simulink model "RR_Aero_Forces"  (R2023b)
settings: Solver=ode45  StartTime=0.0  StopTime=10.0  RelTol=1e-3
values from neighbouring files (symbols this model uses):
  RR_Aero_Aoa = [-40 -20 -10 -5 0 5 10 20 40]    [RR.mat]    (also in aero.m = [-40.0, -20.0, -10.0, -5.0, 0.0, 5.0, 10.0, 20.0, 40.0])
  RR_Aero_CD = [0.682566420597 0.618503123563 0.559439658146 0.524132967178 0.485737326161 0.447874599784 0.410140259349 0.344355457301 0.271986762452 0.285740001736 0.220860646778 0.173194791928 ... (405 elements, 9x9x5)]    [RR.mat]    (also in aero.m = flip([0.271986762452 0.048967807354 0.024623797928 0.0311930)
  RR_Aero_CL = [-1.32787481318 -1.28000797148 -1.22978921447 -1.19580936529 -1.15925228344 -1.11732991534 -1.07321949156 -0.982213833372 -0.840672452343 -1.01110225062 -0.901800471345 -0.804191382013 ... (405 elements, 9x9x5)]    [RR.mat]    (also in aero.m = flip([-0.840672452343 -0.271053660865 0.064194032020 0.23384)
  RR_Aero_CMy = [0.261776710059 0.227892723507 0.194122810948 0.17203964717 0.149197278338 0.123782621534 0.09809104025 0.048156954183 -0.022673613914 0.230490752369 0.172298182326 0.122095577928 ... (405 elements, 9x9x5)]    [RR.mat]    (also in aero.m = flip([-0.022673613914 -0.123256713392 -0.153636001960 -0.164)
  RR_Aero_Elevons = [-40 -20 -10 -5 0 5 10 20 40]    [RR.mat]    (also in aero.m = [-40.0, -20.0, -10.0, -5.0, 0.0, 5.0, 10.0, 20.0, 40.0])
  RR_Aero_Mach = [0.01 0.1 0.2 0.5 0.9]    [RR.mat]    (also in aero.m = [0.01, 0.1, 0.2, 0.5, 0.9])
  RR_Span = 3.6    [RR.mat]
  RR_X_CG = 0.732425    [RR.mat]
  RR_X_NP = 0.9170209    [RR.mat]
libraries: aerolibasang x2, aerolibadyn x1, aerolibatmos2 x1
settings Model: Creator=jrighetti  LastModifiedBy=jrighetti

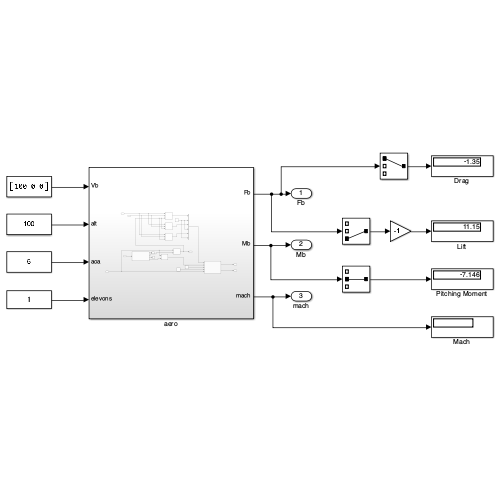
[thumbnail: Simulink's stored preview of the top-level diagram]
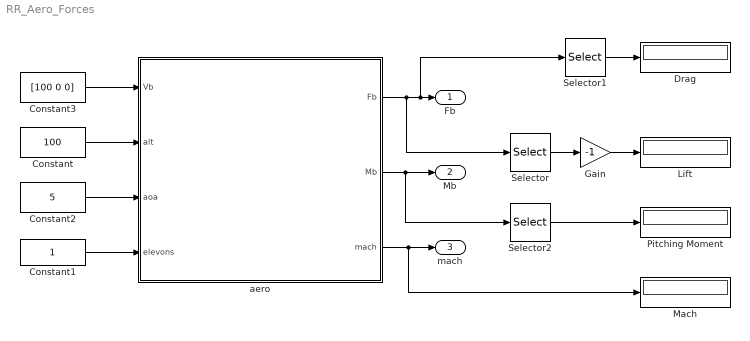
== system RR_Aero_Forces ==
  Constant : Constant  Value=100
  Constant1 : Constant
  Constant2 : Constant  Value=5
  Constant3 : Constant  Value=[100 0 0]
  Drag : Display
  Gain : Gain  Gain=-1
  Lift : Display
  Mach : Display
  Pitching Moment : Display
  Selector : Selector  InputPortWidth=3  IndexOptions=Index vector (dialog)  Indices=[3]  OutputSizes=1
  Selector1 : Selector  InputPortWidth=3  IndexOptions=Index vector (dialog)  Indices=[1]  OutputSizes=1
  Selector2 : Selector  InputPortWidth=3  IndexOptions=Index vector (dialog)  Indices=2  OutputSizes=1
  aero : Subsystem
  Fb : Outport
  Mb : Outport  Port=2
  mach : Outport  Port=3
  wires:
  Constant/1 -> aero/2(alt)
  Constant1/1 -> aero/4(elevons)
  Constant2/1 -> aero/3(aoa)
  Constant3/1 -> aero/1(Vb)
  aero/1(Fb) -> Selector/1, Selector1/1, Fb/1
  Selector/1 -> Gain/1
  Gain/1 -> Lift/1
  aero/3(mach) -> Mach/1, mach/1
  Selector2/1 -> Pitching Moment/1
  aero/2(Mb) -> Selector2/1, Mb/1
  Selector1/1 -> Drag/1

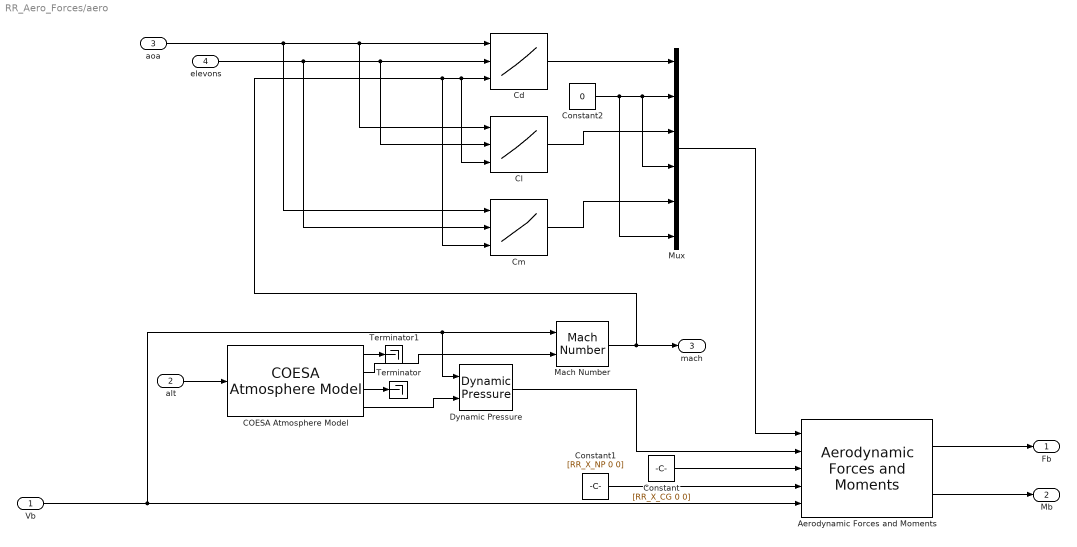
== system RR_Aero_Forces/aero ==
  Vb : Inport
  alt : Inport  Port=2
  aoa : Inport  Port=3
  elevons : Inport  Port=4
  "Aerodynamic Forces and Moments " : aerolibadyn/Aerodynamic Forces and Moments   inputAxes=Wind  outputForceAxes=Body  outputMomentAxes=Body  S=RR_AERO_S  b=RR_Span  cbar=RR_AERO_CORD
  COESA Atmosphere Model : aerolibatmos2/COESA Atmosphere Model  units=English (Velocity in ft/s)  spec=1976 COESA-extended U.S. Standard Atmosphere  model=Profile  profile_var=High temperature  profile_percent=1%  profile_alt=5 km (16404 ft)  envelope_var=High temperature  envelope_percent=1%  action=Warning
  Cd : Lookup_n-D  NumberOfTableDimensions=3  BreakpointsForDimension1=RR_Aero_Aoa  BreakpointsForDimension2=RR_Aero_Elevons  BreakpointsForDimension3=RR_Aero_Mach  BreakpointsForDimension1DataTypeStr=Inherit: Inherit from 'Breakpoint data'  Table=RR_Aero_CD  TableDataTypeStr=Inherit: Inherit from 'Table data'  InternalRulePriority=Speed  RndMeth=Simplest
      settings: InputPortMap=u0,u1,u2
  Cl : Lookup_n-D  NumberOfTableDimensions=3  BreakpointsForDimension1=RR_Aero_Aoa  BreakpointsForDimension2=RR_Aero_Elevons  BreakpointsForDimension3=RR_Aero_Mach  Table=RR_Aero_CL  DiagnosticForOutOfRangeInput=Warning  InternalRulePriority=Speed  RndMeth=Simplest
      settings: InputPortMap=u0,u1,u2
  Cm : Lookup_n-D  NumberOfTableDimensions=3  BreakpointsForDimension1=RR_Aero_Aoa  BreakpointsForDimension2=RR_Aero_Elevons  BreakpointsForDimension3=RR_Aero_Mach  Table=RR_Aero_CMy  DiagnosticForOutOfRangeInput=Warning  InternalRulePriority=Speed  RndMeth=Simplest
      settings: InputPortMap=u0,u1,u2
  Constant : Constant  Value=[RR_X_CG 0 0]
  Constant1 : Constant  Value=[RR_X_NP 0 0]
  Constant2 : Constant  Value=0
  Dynamic Pressure : aerolibasang/Dynamic Pressure
  Mach Number : aerolibasang/Mach Number
  Mux : Mux  Inputs=6
  Terminator : Terminator
  Terminator1 : Terminator
  Fb : Outport
  Mb : Outport  Port=2
  mach : Outport  Port=3
  wires:
  Dynamic Pressure/1 -> "Aerodynamic Forces and Moments "/2
  Constant2/1 -> Mux/6, Mux/4, Mux/2
  alt/1 -> COESA Atmosphere Model/1
  "Aerodynamic Forces and Moments "/1 -> Fb/1
  COESA Atmosphere Model/2 -> Mach Number/2
  COESA Atmosphere Model/3 -> Terminator/1
  Constant/1 -> "Aerodynamic Forces and Moments "/3
  COESA Atmosphere Model/4 -> Dynamic Pressure/2
  "Aerodynamic Forces and Moments "/2 -> Mb/1
  elevons/1 -> Cm/2, Cl/2, Cd/2
  Mach Number/1 -> mach/1, Cm/3, Cl/3, Cd/3
  Mux/1 -> "Aerodynamic Forces and Moments "/1
  Cl/1 -> Mux/3
  Constant1/1 -> "Aerodynamic Forces and Moments "/4
  aoa/1 -> Cm/1, Cl/1, Cd/1
  Cd/1 -> Mux/1
  COESA Atmosphere Model/1 -> Terminator1/1
  Cm/1 -> Mux/5
  Vb/1 -> "Aerodynamic Forces and Moments "/5, Dynamic Pressure/1, Mach Number/1
